simulink model "vehicle_model"  (R2023a)
settings: Solver=VariableStepAuto  StartTime=0.0  StopTime=10.0  RelTol=1e-3
settings Model: Creator=Pedro  LastModifiedBy=Pedro

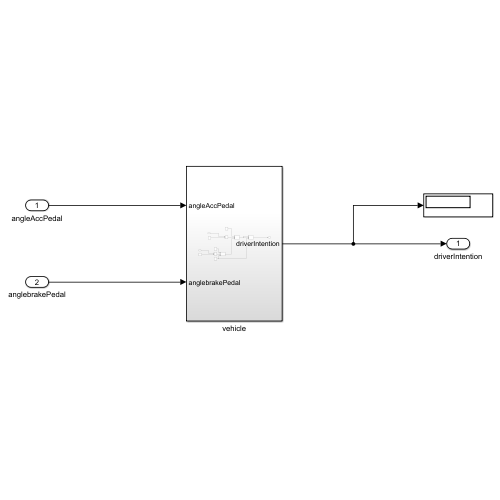
[thumbnail: Simulink's stored preview of the top-level diagram]
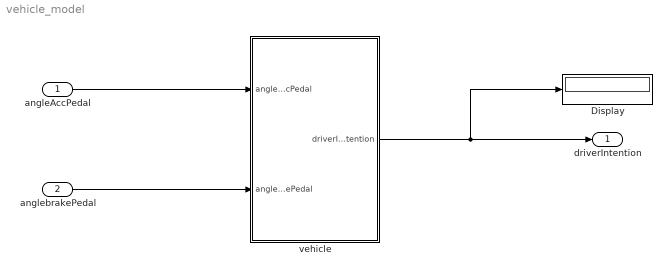
== system vehicle_model ==
  angleAccPedal : Inport
  anglebrakePedal : Inport  Port=2
  Display : Display
  vehicle : Subsystem
  driverIntention : Outport
  wires:
  angleAccPedal/1 -> vehicle/1(angleAccPedal)
  anglebrakePedal/1 -> vehicle/2(anglebrakePedal)
  vehicle/1(driverIntention) -> Display/1, driverIntention/1

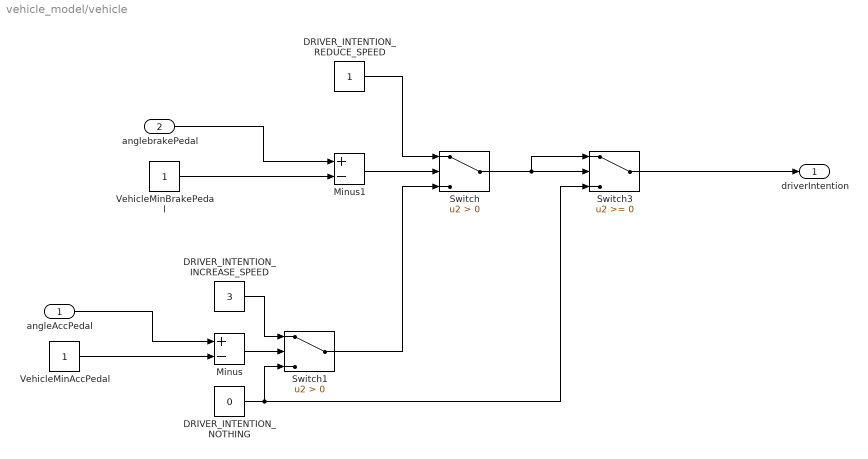
== system vehicle_model/vehicle ==
  angleAccPedal : Inport
  anglebrakePedal : Inport  Port=2
  DRIVER_INTENTION_INCREASE_SPEED : Constant  Value=3
  DRIVER_INTENTION_NOTHING : Constant  Value=0
  DRIVER_INTENTION_REDUCE_SPEED : Constant
  Minus : Sum  Inputs=+-
  Minus1 : Sum  Inputs=+-
  Switch : Switch  Criteria=u2 > Threshold  SaturateOnIntegerOverflow=off  InputSameDT=off
  Switch1 : Switch  Criteria=u2 > Threshold  SaturateOnIntegerOverflow=off  InputSameDT=off
  Switch3 : Switch  SaturateOnIntegerOverflow=off  InputSameDT=off
  VehicleMinAccPedal : Constant
  VehicleMinBrakePedal : Constant
  driverIntention : Outport
  wires:
  DRIVER_INTENTION_NOTHING/1 -> Switch1/3, Switch3/3
  Switch3/1 -> driverIntention/1
  Switch/1 -> Switch3/1, Switch3/2
  Switch1/1 -> Switch/3
  DRIVER_INTENTION_INCREASE_SPEED/1 -> Switch1/1
  VehicleMinBrakePedal/1 -> Minus1/2
  VehicleMinAccPedal/1 -> Minus/2
  Minus/1 -> Switch1/2
  anglebrakePedal/1 -> Minus1/1
  angleAccPedal/1 -> Minus/1
  Minus1/1 -> Switch/2
  DRIVER_INTENTION_REDUCE_SPEED/1 -> Switch/1
